simulink library "carnotUIBK_bus"  (R2023b)
settings: Solver=VariableStepAuto  StartTime=0.0  StopTime=10.0  RelTol=1e-3  EnableMultiTasking=on
values from neighbouring files (symbols this model uses):
  A = 7*10*2    (= 140)    [theta_ground_v1.m]    (also in xlswrite1.m = num2cell(data))
  amb_factor = 1    [DOOR.m]    (also in WALL.m; WINDOW.m = 0)
  area = obj.width * obj.height    [DOOR.m]    (also in RES.m = []; ROOM.m = 0; THERMALZONE.m = area + room(kk).area; WALL.m = area - obj.doors(jj).calc_area())
  B = A/(0.5 * P)    (= 8.23529411765)    [theta_ground_v1.m]
  boundary = BOUNDARY()    [BUILDING.m]    (also in WALL.m = '')
  building = obj    [BUILDING.m]    (also in create_building_automatic.m = building.save(); ini_building_automatic.m = building.add_variant_hvac(building.variant_hvac, hvac); load_building_automatic.m = building.save())
  C = zeros(1,length(d)+1)    [CONSTRUCTION.m]    (also in DOOR.m = [0 0 0]; WALL.m = [0 0 0]; WINDOW.m = [0 0 0])
  control = 2    [GAIN.m]    (also in GAINS.m)
  cp = str2num(value)    [CONSTRUCTION.m]
  height = 0    [DOOR.m]    (also in ROOM.m; THERMALZONE.m; WALL.m; WINDOW.m)
  p = [timevec_weather weather(:,12)]    [BOUNDARY.m]    (also in WEATHER.m = 0; init_carnotUIBK.m = cell2mat(carnotUIBKpaths(i,2)))
  rho = str2num(value)    [CONSTRUCTION.m]    (also in theta_ground_v1.m = 2000)
  type = 1    [CONSTRUCTION.m]    (also in GAINS.m = raw_moisture{ii,3}; STRUCTURE.m = 0)
  view_factor = 1    [DOOR.m]    (also in WINDOW.m = 0)
  wall = []    [ROOM.m]
  z = obj.Z    [WALL.m]    (also in theta_ground_v1.m = 0)
  zone = obj.zone(ind)    [THERMALZONE.m]
undefined symbols (not defined in the file or in its folder): const, Dd, get_building, mdot_air, mdot_CO2, mdot_H2O, mdot_VOC, pos, Qdot_C, Qdot_H, Qdot_I_electricity, Qdot_I_light, Qdot_I_person, Qdot_S, Qdot_T_ground, Qdot_T_internal, Qdot_T_neighbour, Qdot_T_opaque, Qdot_T_window, Qdot_V_infiltration, Qdot_V_mech, Qdot_V_window, Qdotc, Qdotr, r_frame, solar_ratio, solar_ratio1, solar_ratio2, Tc, Tr, Ts, Uvalue, wallsurface, window, window_height, window_heigth, window_width, windowsurface, x_CO2, x_H2O, x_VOC
libraries: $bdroot x134, carnot x87, simulink_extras x14, slpidlib x4, simulink x3
(part 7 of 12)

== system carnotUIBK_bus/window/window_TF_shading/alfa_window_in ==
  note: Convective and radiative heat transfer at the INDOOR SURFACE OF A VERTICAL WINDOW
      | with 1-4 layers (each 3 ... 8 mm thick)
  note: WINDOW = FRAME + GLASS
  note: s: surface
      | c: convective
      | r: radiative
  note: CONVENTION:
      | Qdot > 0 and qdots < 0, if Ts > T (heat flows from wall surface to room node),
      | Qdot < 0 and qdots > 0, if Ts < T (heat flows from room node to wall surface).
  note: (W/m^2)
  Ts2 : Inport
  "[sun_t]" : Inport  Port=2
  "[AIV]" : Inport  Port=3
  WDB : Inport  Port=4
  control : Inport  Port=5
  Bus Assignment2 : BusAssignment  AssignedSignals=Qdotc,Qdotr,Qdot_S
  Bus Selector : BusSelector  OutputSignals=Tc,Tr
  Fcn : Fcn  Expr=1.6*(abs(u(1)-u(2)))^0.3
  Fcn1 : Fcn  Expr=(273.15+u(1))^4-(273.15+u(2))^4
  Mux2 : Mux  Inputs=2
  Mux3 : Mux  Inputs=2
  Product : Product  InputSameDT=on  RndMeth=Zero  SaturateOnIntegerOverflow=on  OutDataTypeStr=Inherit: Same as first input
  Product1 : Product  InputSameDT=on  RndMeth=Zero  SaturateOnIntegerOverflow=on  OutDataTypeStr=Inherit: Same as first input
  S_initialize : $bdroot/general/S_initialize  SystemSampleTime=-1  VariantActivationTime=update diagram  AllowFlexibleInterface=on  Latency=0  AutoFrameSizeCalculation=off
  Sum : Sum  Inputs=+-  InputSameDT=on  SaturateOnIntegerOverflow=on  OutDataTypeStr=Inherit: Same as first input
  Sum2 : Sum  Inputs=--+  InputSameDT=on  SaturateOnIntegerOverflow=on  OutDataTypeStr=Inherit: Same as first input
  emission_in : Gain  Gain=emission_in  SaturateOnIntegerOverflow=on  OutDataTypeStr=Inherit: Same as input  ParamDataTypeStr=Inherit: Same as input
  sigma : Constant  Value=5.67e-8
  surface of window glass : Gain  Gain=(1-frame)*windowsurface  SaturateOnIntegerOverflow=on  OutDataTypeStr=Inherit: Same as input  ParamDataTypeStr=Inherit: Same as input
  surface of window1 : Gain  Gain=windowsurface  SaturateOnIntegerOverflow=on  OutDataTypeStr=Inherit: Same as input  ParamDataTypeStr=Inherit: Same as input
  surface of window2 : Gain  Gain=windowsurface  SaturateOnIntegerOverflow=on  OutDataTypeStr=Inherit: Same as input  ParamDataTypeStr=Inherit: Same as input
  transmission_absorption : Subsystem
  view_factor : Gain  Gain=view_factor  SaturateOnIntegerOverflow=on  OutDataTypeStr=Inherit: Same as input  ParamDataTypeStr=Inherit: Same as input
  qdots2 : Outport  VectorParamsAs1DForOutWhenUnconnected=off
  "[S]" : Outport  Port=2  VectorParamsAs1DForOutWhenUnconnected=off
  wires:
  control/1 -> transmission_absorption/3(control)
  WDB/1 -> transmission_absorption/2(WDB)
  transmission_absorption/1(qdot_abs) -> Sum2/3  "qabs"
  transmission_absorption/2(qdot_sol) -> surface of window glass/1  "qdot_sol (>=0)"
  surface of window glass/1 -> Bus Assignment2/4  "Qdot_sol"
  "[sun_t]"/1 -> transmission_absorption/1(sun_t)
  Product/1 -> Sum2/2, surface of window2/1  "qdotr"
  Sum2/1 -> qdots2/1
  emission_in/1 -> view_factor/1
  sigma/1 -> emission_in/1
  Fcn1/1 -> Product/2
  view_factor/1 -> Product/1
  "[AIV]"/1 -> Bus Selector/1
  Mux3/1 -> Fcn1/1
  Bus Selector/2 -> Mux3/2  "<Tr>"
  Fcn/1 -> Product1/2  "hc"
  Mux2/1 -> Fcn/1
  Sum/1 -> Product1/1  "dTc"
  Ts2/1 -> Sum/1, Mux2/1, Mux3/1  "Ts"
  Bus Selector/1 -> Sum/2, Mux2/2  "<Tc>"
  Product1/1 -> surface of window1/1, Sum2/1  "qdotc"
  S_initialize/1 -> Bus Assignment2/1
  surface of window1/1 -> Bus Assignment2/2  "[Qdotc, Qdotr]"
  surface of window2/1 -> Bus Assignment2/3  "[Qdotc, Qdotr]"
  Bus Assignment2/1 -> "[S]"/1

== system carnotUIBK_bus/window/window_TF_shading/alfa_window_out ==
  note: WINDOW = FRAME + GLASS
  note: Convective and radiative heat transfer at the OUTDOOR SURFACE OF A VERTICAL WINDOW
  note: modified
      | weatherdata
  note: s: surface
      | c: convective
      | r: radiative
      | h: in height
      | t: tilted surface
  note: CONVENTION:
      | qdots < 0, if Ts > T, heat flows from window surface (resp. room node) to ambition,
      | qdots > 0, if Ts < T, heat flows from ambition to window surface (resp. room node).
  WDB : Inport
  g : Inport  Port=2
  Ts1 : Inport  Port=3
  Bus Assignment2 : BusAssignment  AssignedSignals=Qdot_T_window
  Bus Selector : BusSelector  OutputSignals=Temperature_Ambient,Temperature_Sky_Radiation,Wind_Speed
  Bus Selector1 : BusSelector  OutputSignals=Incidence_Angle_sun,Solar_Radiation_direct_surface,Solar_Radiation_diffuse_surface
  Mux1 : Mux  Inputs=2
  Mux2 : Mux  Inputs=2
  Product6 : Product  InputSameDT=on  SaturateOnIntegerOverflow=on  OutDataTypeStr=Inherit: Same as first input
  Product7 : Product  InputSameDT=on  SaturateOnIntegerOverflow=on  OutDataTypeStr=Inherit: Same as first input
  Radiation_on_Inclined_Surface : carnot/Weather/Radiation_on_Inclined_Surface  sky=Perez 1990  reflect=0.2
      settings: SourceProductName=Carnot
  S_initialize : $bdroot/general/S_initialize  SystemSampleTime=-1  VariantActivationTime=update diagram  AllowFlexibleInterface=on  Latency=0  AutoFrameSizeCalculation=off
  Sum : Sum  Inputs=+-  InputSameDT=on  SaturateOnIntegerOverflow=on  OutDataTypeStr=Inherit: Same as first input
  Sum2 : Sum  Inputs=+++  InputSameDT=on  SaturateOnIntegerOverflow=on  OutDataTypeStr=Inherit: Same as first input
  Sum3 : Sum  InputSameDT=on  SaturateOnIntegerOverflow=on  OutDataTypeStr=Inherit: Same as first input
  absorption_out * frame : Gain  Gain=absorption_out * frame  SaturateOnIntegerOverflow=on  OutDataTypeStr=Inherit: Same as input  ParamDataTypeStr=Inherit: Same as input
  alfa : Fcn  Expr=3*u(1)+2.8
  position : Constant  Value=pos
  qp rad : Subsystem
  surface of window : Gain  Gain=windowsurface  SaturateOnIntegerOverflow=on  OutDataTypeStr=Inherit: Same as input  ParamDataTypeStr=Inherit: Same as input
  "[sun_t]" : Outport  InitialOutput=0  VectorParamsAs1DForOutWhenUnconnected=off
  qdots1 : Outport  Port=2  InitialOutput=0  VectorParamsAs1DForOutWhenUnconnected=off
  "[S]" : Outport  Port=3  InitialOutput=0  VectorParamsAs1DForOutWhenUnconnected=off
  wires:
  Radiation_on_Inclined_Surface/1 -> Bus Selector1/1
  position/1 -> Radiation_on_Inclined_Surface/2
  Product7/1 -> Sum2/1  "qdot,conv"
  alfa/1 -> Product7/2  "alfa"
  qp rad/1(qprad) -> Sum2/2  "qdotr"
  Ts1/1 -> qp rad/2(Tw), Sum/2  "Ts (outer wall surface)"
  Mux1/1 -> "[sun_t]"/1
  Bus Selector1/2 -> Mux2/1, Sum3/1  "<Solar_Radiation_direct_surface>"
  absorption_out * frame/1 -> Sum2/3
  g/1 -> Product6/2
  Sum2/1 -> surface of window/1, qdots1/1
  Sum3/1 -> absorption_out * frame/1
  Bus Selector1/1 -> Mux1/1  "<Incidence_Angle_sun>"
  WDB/1 -> Radiation_on_Inclined_Surface/1, Bus Selector/1
  Sum/1 -> Product7/1  "dTc"
  Product6/1 -> Mux1/2
  Mux2/1 -> Product6/1
  Bus Selector1/3 -> Mux2/2, Sum3/2  "<Solar_Radiation_diffuse_surface>"
  Bus Selector/1 -> qp rad/1(Ta), Sum/1  "<Temperature_Ambient>"
  Bus Selector/2 -> qp rad/3(Tsky)  "<Temperature_Sky_Radiation>"
  Bus Selector/3 -> alfa/1  "<Wind_Speed>"
  Bus Assignment2/1 -> "[S]"/1
  surface of window/1 -> Bus Assignment2/2
  S_initialize/1 -> Bus Assignment2/1

== system carnotUIBK_bus/window/window_TF_shading/lambda_window ==
  note: Heat conduction in a window (ONLY SURFACE LAYER CONNECTABLE)
  note: Timeconstant of window is calculated
      | in the mask initialization
  qdots1 : Inport
  qdots2 : Inport  Port=2
  Product1 : Product  InputSameDT=on  RndMeth=Zero  SaturateOnIntegerOverflow=on  OutDataTypeStr=Inherit: Same as first input
  Product6 : Product  InputSameDT=on  RndMeth=Zero  SaturateOnIntegerOverflow=on  OutDataTypeStr=Inherit: Same as first input
  R_win : Constant  Value=Rwin
  Sum1 : Sum  InputSameDT=on  SaturateOnIntegerOverflow=on  OutDataTypeStr=Inherit: Same as first input
  Sum3 : Sum  InputSameDT=on  SaturateOnIntegerOverflow=on  OutDataTypeStr=Inherit: Same as first input
  Transfer Fcn : TransferFcn  Denominator=[timeconst 1]
  Transfer Fcn1 : TransferFcn  Denominator=[timeconst 1]
  Ts1 : Outport  VectorParamsAs1DForOutWhenUnconnected=off
  Ts2 : Outport  Port=2  VectorParamsAs1DForOutWhenUnconnected=off
  wires:
  Transfer Fcn1/1 -> Ts2/1, Sum3/2
  Transfer Fcn/1 -> Ts1/1, Sum1/2
  qdots1/1 -> Product6/2
  qdots2/1 -> Product1/2
  Product6/1 -> Sum3/1
  Sum3/1 -> Transfer Fcn/1
  Product1/1 -> Sum1/1
  Sum1/1 -> Transfer Fcn1/1
  R_win/1 -> Product6/1, Product1/1  "R_win"

== system carnotUIBK_bus/HVAC/HVAC_1001_electrical heaters/electrical heater zone 1/Transfer Fcn (with initial states) ==
  In1 : Inport
  State Space : StateSpace  A=A  B=B  C=C  D=Dd  InitialCondition=X0
  Out1 : Outport  InitialOutput=0  VectorParamsAs1DForOutWhenUnconnected=off
  wires:
  In1/1 -> State Space/1
  State Space/1 -> Out1/1

== system carnotUIBK_bus/HVAC/HVAC_2001_ventilation system simple/ventilation_zone 1/Subsystem ==
  note: (kg/s)
  note: (kg/s)
  note: (kg/s)
  note: (kg/kg)
  note: (kg/kg)
  note: ASSUMPTION: mdot_air_out2in = mdot_air_in2out !
  mdot_air : Inport
  x_in : Inport  Port=2
  x_out : Inport  Port=3
  Demux2 : Demux  Outputs=2
      settings: DisplayOption=none
  Demux3 : Demux  Outputs=2
      settings: DisplayOption=none
  Fcn{,1..3} (4 alike) : Fcn  Expr=u / (1+u)
  Product5 : Product  InputSameDT=on  SaturateOnIntegerOverflow=on  OutDataTypeStr=Inherit: Same as first input
  Product6 : Product  InputSameDT=on  SaturateOnIntegerOverflow=on  OutDataTypeStr=Inherit: Same as first input
  Sum1 : Sum  Inputs=+-  InputSameDT=on  SaturateOnIntegerOverflow=on  OutDataTypeStr=Inherit: Same as first input
  Sum2 : Sum  Inputs=+-  InputSameDT=on  SaturateOnIntegerOverflow=on  OutDataTypeStr=Inherit: Same as first input
  mdot_H2O : Outport  VectorParamsAs1DForOutWhenUnconnected=off
  mdot_CO2 : Outport  Port=2  VectorParamsAs1DForOutWhenUnconnected=off
  wires:
  x_out/1 -> Demux2/1
  Demux2/1 -> Fcn/1  "x_H2O_out"
  Demux2/2 -> Fcn1/1  "x_CO2_out"
  Demux3/2 -> Fcn3/1  "x_CO2_in"
  Demux3/1 -> Fcn2/1  "x_H2O_in"
  x_in/1 -> Demux3/1
  Fcn/1 -> Sum1/1
  Fcn2/1 -> Sum1/2
  Fcn1/1 -> Sum2/1
  Fcn3/1 -> Sum2/2
  Sum2/1 -> Product6/2
  Sum1/1 -> Product5/2
  mdot_air/1 -> Product6/1, Product5/1  "mdot_air >=0"
  Product6/1 -> mdot_CO2/1
  Product5/1 -> mdot_H2O/1

== system carnotUIBK_bus/HVAC/HVAC_9002_window opening/window opening 1/Transfer Fcn (with initial states) ==
  In1 : Inport
  State Space : StateSpace  A=A  B=B  C=C  D=Dd  InitialCondition=X0
  Out1 : Outport  InitialOutput=0  VectorParamsAs1DForOutWhenUnconnected=off
  wires:
  In1/1 -> State Space/1
  State Space/1 -> Out1/1

== system carnotUIBK_bus/HVAC/HVAC_9002_window opening/window opening 1/Transfer Fcn (with initial states)1 ==
  In1 : Inport
  State Space : StateSpace  A=A  B=B  C=C  D=Dd  InitialCondition=X0
  Out1 : Outport  InitialOutput=0  VectorParamsAs1DForOutWhenUnconnected=off
  wires:
  State Space/1 -> Out1/1
  In1/1 -> State Space/1

== system carnotUIBK_bus/HVAC/HVAC_9002_window opening/window opening 1/Transfer Fcn (with initial states)2 ==
  In1 : Inport
  State Space : StateSpace  A=A  B=B  C=C  D=Dd  InitialCondition=X0
  Out1 : Outport  InitialOutput=0  VectorParamsAs1DForOutWhenUnconnected=off
  wires:
  In1/1 -> State Space/1
  State Space/1 -> Out1/1

== system carnotUIBK_bus/HVAC/HVAC_9002_window opening/window opening 2/Transfer Fcn (with initial states)1 ==
  In1 : Inport
  State Space : StateSpace  A=A  B=B  C=C  D=Dd  InitialCondition=X0
  Out1 : Outport  InitialOutput=0  VectorParamsAs1DForOutWhenUnconnected=off
  wires:
  State Space/1 -> Out1/1
  In1/1 -> State Space/1

== system carnotUIBK_bus/HVAC/HVAC_9002_window opening/window opening 2/Transfer Fcn (with initial states)2 ==
  In1 : Inport
  State Space : StateSpace  A=A  B=B  C=C  D=Dd  InitialCondition=X0
  Out1 : Outport  InitialOutput=0  VectorParamsAs1DForOutWhenUnconnected=off
  wires:
  In1/1 -> State Space/1
  State Space/1 -> Out1/1

== system carnotUIBK_bus/HVAC/HVAC_9002_window opening/window opening 2/Transfer Fcn (with initial states)3 ==
  In1 : Inport
  State Space : StateSpace  A=A  B=B  C=C  D=Dd  InitialCondition=X0
  Out1 : Outport  InitialOutput=0  VectorParamsAs1DForOutWhenUnconnected=off
  wires:
  In1/1 -> State Space/1
  State Space/1 -> Out1/1

== system carnotUIBK_bus/HVAC/HVAC_9002_window opening/window opening 3/Transfer Fcn (with initial states)1 ==
  In1 : Inport
  State Space : StateSpace  A=A  B=B  C=C  D=Dd  InitialCondition=X0
  Out1 : Outport  InitialOutput=0  VectorParamsAs1DForOutWhenUnconnected=off
  wires:
  State Space/1 -> Out1/1
  In1/1 -> State Space/1

== system carnotUIBK_bus/HVAC/HVAC_9002_window opening/window opening 3/Transfer Fcn (with initial states)2 ==
  In1 : Inport
  State Space : StateSpace  A=A  B=B  C=C  D=Dd  InitialCondition=X0
  Out1 : Outport  InitialOutput=0  VectorParamsAs1DForOutWhenUnconnected=off
  wires:
  In1/1 -> State Space/1
  State Space/1 -> Out1/1

== system carnotUIBK_bus/HVAC/HVAC_9002_window opening/window opening 3/Transfer Fcn (with initial states)3 ==
  In1 : Inport
  State Space : StateSpace  A=A  B=B  C=C  D=Dd  InitialCondition=X0
  Out1 : Outport  InitialOutput=0  VectorParamsAs1DForOutWhenUnconnected=off
  wires:
  In1/1 -> State Space/1
  State Space/1 -> Out1/1

== system carnotUIBK_bus/HVAC/HVAC_9002_window opening/window opening 4/Transfer Fcn (with initial states)1 ==
  In1 : Inport
  State Space : StateSpace  A=A  B=B  C=C  D=Dd  InitialCondition=X0
  Out1 : Outport  InitialOutput=0  VectorParamsAs1DForOutWhenUnconnected=off
  wires:
  State Space/1 -> Out1/1
  In1/1 -> State Space/1

== system carnotUIBK_bus/HVAC/HVAC_9002_window opening/window opening 4/Transfer Fcn (with initial states)2 ==
  In1 : Inport
  State Space : StateSpace  A=A  B=B  C=C  D=Dd  InitialCondition=X0
  Out1 : Outport  InitialOutput=0  VectorParamsAs1DForOutWhenUnconnected=off
  wires:
  In1/1 -> State Space/1
  State Space/1 -> Out1/1

== system carnotUIBK_bus/HVAC/HVAC_9002_window opening/window opening 4/Transfer Fcn (with initial states)3 ==
  In1 : Inport
  State Space : StateSpace  A=A  B=B  C=C  D=Dd  InitialCondition=X0
  Out1 : Outport  InitialOutput=0  VectorParamsAs1DForOutWhenUnconnected=off
  wires:
  In1/1 -> State Space/1
  State Space/1 -> Out1/1

== system carnotUIBK_bus/HVAC/HVAC_9002_window opening/window opening 5/Transfer Fcn (with initial states)1 ==
  In1 : Inport
  State Space : StateSpace  A=A  B=B  C=C  D=Dd  InitialCondition=X0
  Out1 : Outport  InitialOutput=0  VectorParamsAs1DForOutWhenUnconnected=off
  wires:
  State Space/1 -> Out1/1
  In1/1 -> State Space/1

== system carnotUIBK_bus/HVAC/HVAC_9002_window opening/window opening 5/Transfer Fcn (with initial states)2 ==
  In1 : Inport
  State Space : StateSpace  A=A  B=B  C=C  D=Dd  InitialCondition=X0
  Out1 : Outport  InitialOutput=0  VectorParamsAs1DForOutWhenUnconnected=off
  wires:
  In1/1 -> State Space/1
  State Space/1 -> Out1/1

== system carnotUIBK_bus/HVAC/HVAC_9002_window opening/window opening 5/Transfer Fcn (with initial states)3 ==
  In1 : Inport
  State Space : StateSpace  A=A  B=B  C=C  D=Dd  InitialCondition=X0
  Out1 : Outport  InitialOutput=0  VectorParamsAs1DForOutWhenUnconnected=off
  wires:
  In1/1 -> State Space/1
  State Space/1 -> Out1/1

== system carnotUIBK_bus/HVAC/HVAC_9002_window opening/window opening 6/Transfer Fcn (with initial states)1 ==
  In1 : Inport
  State Space : StateSpace  A=A  B=B  C=C  D=Dd  InitialCondition=X0
  Out1 : Outport  InitialOutput=0  VectorParamsAs1DForOutWhenUnconnected=off
  wires:
  State Space/1 -> Out1/1
  In1/1 -> State Space/1

== system carnotUIBK_bus/HVAC/HVAC_9002_window opening/window opening 6/Transfer Fcn (with initial states)2 ==
  In1 : Inport
  State Space : StateSpace  A=A  B=B  C=C  D=Dd  InitialCondition=X0
  Out1 : Outport  InitialOutput=0  VectorParamsAs1DForOutWhenUnconnected=off
  wires:
  In1/1 -> State Space/1
  State Space/1 -> Out1/1

== system carnotUIBK_bus/HVAC/HVAC_9002_window opening/window opening 6/Transfer Fcn (with initial states)3 ==
  In1 : Inport
  State Space : StateSpace  A=A  B=B  C=C  D=Dd  InitialCondition=X0
  Out1 : Outport  InitialOutput=0  VectorParamsAs1DForOutWhenUnconnected=off
  wires:
  In1/1 -> State Space/1
  State Space/1 -> Out1/1

== system carnotUIBK_bus/gain/People/W//ppl (activity)/LUT_Qdot_dry ==
  note: SENSITIVE/DRY HEAT POWER emitted from a person in a room
  activity : Inport
  Top : Inport  Port=2
  Look-Up Table Qdot_dry : Subsystem  mask(Lookup Table (2-D)){x=[10 12 14 16 18 20 22 23 24 25 26 28 30 32 34], y=[0 1 2 3 4], t=[135 135 135 170 210; 125 125 125 160 195; 115 115 115 150 180; 105 105 105 135 165; 100 100 100 125 152; 95 95 95 115 140; 90 90 90 105 125; 85 85 85 100 117; 80 80 80 95 110; 75 75 75 90 102; 70 70 70 85 95; 60 60 60 70 80; 50 50 50 60 65; 30 30 30 35 40; 0 0 0 0 0]}
      mask prompts: x "Row:"; y "Column:"; t "Table:"
      mask help: Performs 2-D linear interpolation of input values using the specified input/output table. Extrapolation is performed outside the table boundaries.
      mask init:
      | [r,c]=size(t);
      | x=reshape(x,prod(size(x)),1);
      | xi=x(:,ones(1,c));
      | minx=min(x); maxx=max(x);
      | mint=min(min(t)); maxt=max(max(t));
      mask Display: plot(xi,t,[minx maxx],[mint mint],[minx minx],[mint maxt])
  Qdot_dry : Outport  InitialOutput=0  VectorParamsAs1DForOutWhenUnconnected=off
  wires:
  activity/1 -> Look-Up Table Qdot_dry/2(Cols)
  Look-Up Table Qdot_dry/1(U) -> Qdot_dry/1
  Top/1 -> Look-Up Table Qdot_dry/1(Rows)

== system carnotUIBK_bus/gain/People/W//ppl (activity)/LUT_Qdot_hum1 ==
  note: LATENT/HUMID HEAT POWER emitted from a person in a room
  activity : Inport
  Top : Inport  Port=2
  Look-Up Table Qdot_hum : Subsystem  mask(Lookup Table (2-D)){x=[10 12 14 16 18 20 22 23 24 25 26 28 30 32 34], y=[0 1 2 3 4], t=[20 20 20 55 100; 20 20 20 55 100; 20 20 20 55 100; 21 21 21 58 105; 23 23 23 65 115; 25 25 25 75 130; 30 30 30 85 145; 35 35 35 90 155; 40 40 40 95 160; 45 45 45 100 167; 50 50 50 105 175; 60 60 60 115 190; 70 70 70 125 205; 80 80 80 135 225; 90 90 90 145 245]}
      mask prompts: x "Row:"; y "Column:"; t "Table:"
      mask help: Performs 2-D linear interpolation of input values using the specified input/output table. Extrapolation is performed outside the table boundaries.
      mask init:
      | [r,c]=size(t);
      | x=reshape(x,prod(size(x)),1);
      | xi=x(:,ones(1,c));
      | minx=min(x); maxx=max(x);
      | mint=min(min(t)); maxt=max(max(t));
      mask Display: plot(xi,t,[minx maxx],[mint mint],[minx minx],[mint maxt])
  Qdot_hum : Outport  InitialOutput=0  VectorParamsAs1DForOutWhenUnconnected=off
  wires:
  Top/1 -> Look-Up Table Qdot_hum/1(Rows)
  activity/1 -> Look-Up Table Qdot_hum/2(Cols)
  Look-Up Table Qdot_hum/1(U) -> Qdot_hum/1

== system carnotUIBK_bus/gain/People/W//ppl (activity)/LUT_mdot_CO2 ==
  note: CO2 MASS FLOW emitted from a person in a room
  activity : Inport
  Look-Up mdot_CO2 : Lookup  InputValues=[0 1 2 3 4]  Table=[0.567 0.708 1.133 2.031 3.305]*10^-5
  mdot_CO2 : Outport  InitialOutput=0  VectorParamsAs1DForOutWhenUnconnected=off
  wires:
  Look-Up mdot_CO2/1 -> mdot_CO2/1
  activity/1 -> Look-Up mdot_CO2/1

== system carnotUIBK_bus/gain/People/W//ppl (activity)/LUT_mdot_H2O ==
  note: WATER MASS FLOW emitted from a person in a room
  activity : Inport
  Top : Inport  Port=2
  Look-Up Table mdot_H2O : Subsystem  mask(Lookup Table (2-D)){x=[10 12 14 16 18 20 22 23 24 25 26 32], y=[0 1 2 3 4], t=[30 30 30 90 150; 30 30 30 90 150; 30 30 30 90 150; 30 30 30 90 155; 35 35 35 95 165; 40 40 40 110 185; 45 45 45 125 200; 50 50 50 130 210; 55 55 55 130 225; 60 60 60 140 240; 65 65 65 150 270; 120 120 120 250 450]/(3.6*1e6)}
      mask prompts: x "Row:"; y "Column:"; t "Table:"
      mask help: Performs 2-D linear interpolation of input values using the specified input/output table. Extrapolation is performed outside the table boundaries.
      mask init:
      | [r,c]=size(t);
      | x=reshape(x,prod(size(x)),1);
      | xi=x(:,ones(1,c));
      | minx=min(x); maxx=max(x);
      | mint=min(min(t)); maxt=max(max(t));
      mask Display: plot(xi,t,[minx maxx],[mint mint],[minx minx],[mint maxt])
  mdot_H2O : Outport  InitialOutput=0  VectorParamsAs1DForOutWhenUnconnected=off
  wires:
  Look-Up Table mdot_H2O/1(U) -> mdot_H2O/1
  activity/1 -> Look-Up Table mdot_H2O/2(Cols)
  Top/1 -> Look-Up Table mdot_H2O/1(Rows)

== system carnotUIBK_bus/gain/People/W//ppl (constant)/LUT_mdot_CO2 ==
  note: CO2 MASS FLOW emitted from a person in a room
  activity : Inport
  Look-Up mdot_CO2 : Lookup  InputValues=[0 1 2 3 4]  Table=[0.567 0.708 1.133 2.031 3.305]*10^-5
  mdot_CO2 : Outport  InitialOutput=0  VectorParamsAs1DForOutWhenUnconnected=off
  wires:
  Look-Up mdot_CO2/1 -> mdot_CO2/1
  activity/1 -> Look-Up mdot_CO2/1

== system carnotUIBK_bus/gain/People/W//ppl (constant)/LUT_mdot_H2O ==
  note: WATER MASS FLOW emitted from a person in a room
  activity : Inport
  Top : Inport  Port=2
  Look-Up Table mdot_H2O : Subsystem  mask(Lookup Table (2-D)){x=[10 12 14 16 18 20 22 23 24 25 26 32], y=[0 1 2 3 4], t=[30 30 30 90 150; 30 30 30 90 150; 30 30 30 90 150; 30 30 30 90 155; 35 35 35 95 165; 40 40 40 110 185; 45 45 45 125 200; 50 50 50 130 210; 55 55 55 130 225; 60 60 60 140 240; 65 65 65 150 270; 120 120 120 250 450]/(3.6*1e6)}
      mask prompts: x "Row:"; y "Column:"; t "Table:"
      mask help: Performs 2-D linear interpolation of input values using the specified input/output table. Extrapolation is performed outside the table boundaries.
      mask init:
      | [r,c]=size(t);
      | x=reshape(x,prod(size(x)),1);
      | xi=x(:,ones(1,c));
      | minx=min(x); maxx=max(x);
      | mint=min(min(t)); maxt=max(max(t));
      mask Display: plot(xi,t,[minx maxx],[mint mint],[minx minx],[mint maxt])
  mdot_H2O : Outport  InitialOutput=0  VectorParamsAs1DForOutWhenUnconnected=off
  wires:
  Look-Up Table mdot_H2O/1(U) -> mdot_H2O/1
  activity/1 -> Look-Up Table mdot_H2O/2(Cols)
  Top/1 -> Look-Up Table mdot_H2O/1(Rows)

== system carnotUIBK_bus/infiltration/infiltration_pressure/infiltration_pressure/dP_infiltration ==
  T_int : Inport
  T_ext : Inport  Port=2
  windspeed : Inport  Port=3
  wind_angle : Inport  Port=4
  air_density_ext : Inport  Port=5
  H_window : Inport  Port=6
  add_coeff_wind : Inport  Port=7
  facade_angle : Inport  Port=8
  Add : Sum
  Add1 : Sum
  Divide : Product  Inputs=/****
  Gain : Gain  Gain=0.5
  K : Constant  Value=273.15
  Product : Product
  Product1 : Product  Inputs=3
  Sum : Sum  Inputs=|+-
  calculate wind_coeff : Subsystem
  g : Constant  Value=9.81
  half of window height : Gain  Gain=0.5
  dP_total : Outport  VectorParamsAs1DForOutWhenUnconnected=off
  wires:
  T_int/1 -> Add1/2, Sum/1
  T_ext/1 -> Sum/2
  Sum/1 -> Divide/2  "delta_T"
  air_density_ext/1 -> Product1/1, Divide/4
  Product/1 -> Gain/1
  Gain/1 -> Product1/3
  Add/1 -> dP_total/1
  g/1 -> Divide/3
  half of window height/1 -> Divide/5
  H_window/1 -> half of window height/1
  wind_angle/1 -> calculate wind_coeff/1(wind_angle)
  calculate wind_coeff/1(wind_coeff) -> Product1/2
  add_coeff_wind/1 -> calculate wind_coeff/2(additional_coeff_wind)
  facade_angle/1 -> calculate wind_coeff/3(facade_angle)
  Product1/1 -> Add/2
  windspeed/1 -> Product/1, Product/2
  Divide/1 -> Add/1
  K/1 -> Add1/1
  Add1/1 -> Divide/1

== system carnotUIBK_bus/infiltration/infiltration_pressure/infiltration_pressure/power_law_infiltration ==
  dP : Inport
  C : Inport  Port=2
  n : Inport  Port=3
  density : Inport  Port=4
  1/3600 : Gain  Gain=1/3600
  Product2 : Product
  Product4 : Product
  abs : Abs  SaturateOnIntegerOverflow=off
  pow_law : Math  Operator=pow  SignedPower=on
  m_dot : Outport  VectorParamsAs1DForOutWhenUnconnected=off
  wires:
  pow_law/1 -> Product2/1
  C/1 -> 1/3600/1
  Product2/1 -> Product4/1
  n/1 -> pow_law/2
  dP/1 -> abs/1
  density/1 -> Product4/2
  Product4/1 -> m_dot/1
  1/3600/1 -> Product2/2
  abs/1 -> pow_law/1

== system carnotUIBK_bus/room_node/1-node/pressure/Subsystem ==
  note: (J/(kg*K)
  T : Inport
  Celsius2Kelvin : Bias  Bias=273.15  SaturateOnIntegerOverflow=off
  air_gas_constant : Gain  Gain=287  SaturateOnIntegerOverflow=on  OutDataTypeStr=Inherit: Same as input  ParamDataTypeStr=Inherit: Same as input
  R*T ' : Outport  VectorParamsAs1DForOutWhenUnconnected=off
  wires:
  Celsius2Kelvin/1 -> air_gas_constant/1
  T/1 -> Celsius2Kelvin/1
  air_gas_constant/1 -> R*T '/1

== system carnotUIBK_bus/room_node/1-node/pressure/Transfer Fcn (with initial outputs)1 ==
  In1 : Inport
  State Space : StateSpace  A=A  B=B  C=C  D=Dd  InitialCondition=X0
  Out1 : Outport  InitialOutput=0  VectorParamsAs1DForOutWhenUnconnected=off
  wires:
  State Space/1 -> Out1/1
  In1/1 -> State Space/1

== system carnotUIBK_bus/room_node/2-node/density and capacity/Transfer Fcn (with initial outputs) ==
  In1 : Inport
  State Space : StateSpace  A=A  B=B  C=C  D=Dd  InitialCondition=X0
  Out1 : Outport  InitialOutput=0  VectorParamsAs1DForOutWhenUnconnected=off
  wires:
  In1/1 -> State Space/1
  State Space/1 -> Out1/1

== system carnotUIBK_bus/room_node/2-node/pressure/Subsystem ==
  note: (J/(kg*K)
  T : Inport
  Celsius2Kelvin : Bias  Bias=273.15  SaturateOnIntegerOverflow=off
  air_gas_constant : Gain  Gain=287  SaturateOnIntegerOverflow=on  OutDataTypeStr=Inherit: Same as input  ParamDataTypeStr=Inherit: Same as input
  R*T ' : Outport  VectorParamsAs1DForOutWhenUnconnected=off
  wires:
  Celsius2Kelvin/1 -> air_gas_constant/1
  T/1 -> Celsius2Kelvin/1
  air_gas_constant/1 -> R*T '/1

== system carnotUIBK_bus/room_node/2-node/pressure/Transfer Fcn (with initial outputs)1 ==
  In1 : Inport
  State Space : StateSpace  A=A  B=B  C=C  D=Dd  InitialCondition=X0
  Out1 : Outport  InitialOutput=0  VectorParamsAs1DForOutWhenUnconnected=off
  wires:
  State Space/1 -> Out1/1
  In1/1 -> State Space/1

== system carnotUIBK_bus/room_node/2-node_ideal/pressure/Subsystem ==
  note: (J/(kg*K)
  T : Inport
  Celsius2Kelvin : Bias  Bias=273.15  SaturateOnIntegerOverflow=off
  air_gas_constant : Gain  Gain=287  SaturateOnIntegerOverflow=on  OutDataTypeStr=Inherit: Same as input  ParamDataTypeStr=Inherit: Same as input
  R*T ' : Outport  VectorParamsAs1DForOutWhenUnconnected=off
  wires:
  Celsius2Kelvin/1 -> air_gas_constant/1
  T/1 -> Celsius2Kelvin/1
  air_gas_constant/1 -> R*T '/1

== system carnotUIBK_bus/room_node/2-node_ideal/pressure/Transfer Fcn (with initial outputs)1 ==
  In1 : Inport
  State Space : StateSpace  A=A  B=B  C=C  D=Dd  InitialCondition=X0
  Out1 : Outport  InitialOutput=0  VectorParamsAs1DForOutWhenUnconnected=off
  wires:
  State Space/1 -> Out1/1
  In1/1 -> State Space/1

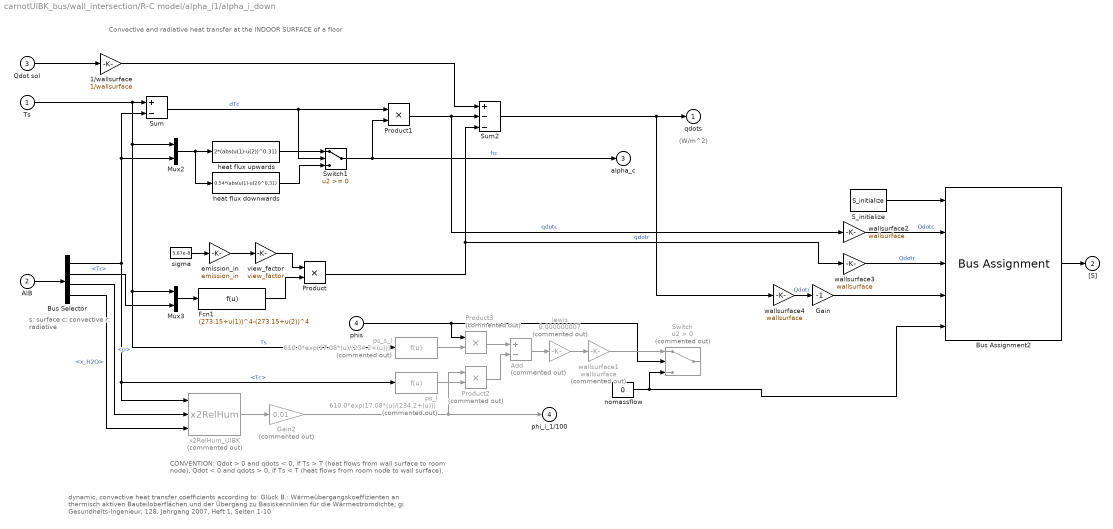
== system carnotUIBK_bus/wall_intersection/R-C model/alpha_i1/alpha_i_down ==
  note: dynamic, convective heat transfer coefficients according to: Glück B.: Wärmeübergangskoeffizienten an thermisch aktiven Bauteiloberflächen
      | und der Übergang zu Basiskennlinien für die Wärmestromdichte; gi Gesundheits-Ingenieur; 128. Jahrgang 2007, Heft 1, Seiten 1-10
  note: s: surface
      | c: convective
      | r: radiative
  note: CONVENTION:
      | Qdot > 0 and qdots < 0, if Ts > T (heat flows from wall surface to room node),
      | Qdot < 0 and qdots > 0, if Ts < T (heat flows from room node to wall surface).
  note: Convective and radiative heat transfer at the INDOOR SURFACE of a floor
  note: (W/m^2)
  Ts : Inport
  AIB : Inport  Port=2
  Qdot sol : Inport  Port=3
  phis : Inport  Port=4
  1/wallsurface : Gain  Gain=1/wallsurface  SaturateOnIntegerOverflow=on  OutDataTypeStr=Inherit: Same as input  ParamDataTypeStr=Inherit: Same as input
  Add : Sum  Commented=on  Inputs=+-
  Bus Assignment2 : BusAssignment  AssignedSignals=Qdotc,Qdotr,Qdot_T_neighbour,mdot_H2O
  Bus Selector : BusSelector  OutputSignals=Tc,Tr,p,x_H2O
  Fcn1 : Fcn  Expr=(273.15+u(1))^4-(273.15+u(2))^4
  Gain : Gain  Gain=-1
  Gain2 : Gain  Commented=on  Gain=0.01
  Mux2 : Mux  Inputs=2
  Mux3 : Mux  Inputs=2
  Product : Product  InputSameDT=on  RndMeth=Zero  SaturateOnIntegerOverflow=on  OutDataTypeStr=Inherit: Same as first input
  Product1 : Product  InputSameDT=on  RndMeth=Zero  SaturateOnIntegerOverflow=on  OutDataTypeStr=Inherit: Same as first input
  Product2 : Product  Commented=on  RndMeth=Zero
  Product3 : Product  Commented=on  RndMeth=Zero
  S_initialize : $bdroot/general/S_initialize  SystemSampleTime=-1  VariantActivationTime=update diagram  AllowFlexibleInterface=on  Latency=0  AutoFrameSizeCalculation=off
  Sum : Sum  Inputs=+-  InputSameDT=on  SaturateOnIntegerOverflow=on  OutDataTypeStr=Inherit: Same as first input
  Sum2 : Sum  Inputs=+--  InputSameDT=on  SaturateOnIntegerOverflow=on  OutDataTypeStr=Inherit: Same as first input
  Switch : Switch  Commented=on  Criteria=u2 > Threshold  SaturateOnIntegerOverflow=off  InputSameDT=off
  Switch1 : Switch  SaturateOnIntegerOverflow=off  InputSameDT=off
  emission_in : Gain  Gain=emission_in  SaturateOnIntegerOverflow=on  OutDataTypeStr=Inherit: Same as input  ParamDataTypeStr=Inherit: Same as input
  heat flux downwards : Fcn  Expr=0.54*(abs(u(1)-u(2))^0.31)
  heat flux upwards : Fcn  Expr=2*(abs(u(1)-u(2))^0.31)
  lewis : Gain  Commented=on  Gain=0.000000007  SaturateOnIntegerOverflow=on  OutDataTypeStr=Inherit: Same as input  ParamDataTypeStr=Inherit: Same as input
  nomassflow : Constant  Value=0
  ps_l : Fcn  Commented=on  Expr=610.0*exp(17.08*(u)/(234.2+(u)))
  ps_s_l : Fcn  Commented=on  Expr=610.0*exp(17.08*(u)/(234.2+(u)))
  sigma : Constant  Value=5.67e-8
  view_factor : Gain  Gain=view_factor  SaturateOnIntegerOverflow=on  OutDataTypeStr=Inherit: Same as input  ParamDataTypeStr=Inherit: Same as input
  wallsurface1 : Gain  Commented=on  Gain=wallsurface  SaturateOnIntegerOverflow=on  OutDataTypeStr=Inherit: Same as input  ParamDataTypeStr=Inherit: Same as input
  wallsurface2 : Gain  Gain=wallsurface  SaturateOnIntegerOverflow=on  OutDataTypeStr=Inherit: Same as input  ParamDataTypeStr=Inherit: Same as input
  wallsurface3 : Gain  Gain=wallsurface  SaturateOnIntegerOverflow=on  OutDataTypeStr=Inherit: Same as input  ParamDataTypeStr=Inherit: Same as input
  wallsurface4 : Gain  Gain=wallsurface  SaturateOnIntegerOverflow=on  OutDataTypeStr=Inherit: Same as input  ParamDataTypeStr=Inherit: Same as input
  x2RelHum_UIBK : carnot/Basic/Material_Properties/x2RelHum  Commented=on
      settings: SourceProductName=Carnot
  qdots : Outport  InitialOutput=0  VectorParamsAs1DForOutWhenUnconnected=off
  "[S]" : Outport  Port=2  InitialOutput=0  VectorParamsAs1DForOutWhenUnconnected=off
  alpha_c : Outport  Port=3  InitialOutput=0  VectorParamsAs1DForOutWhenUnconnected=off
  phi_i_1/100 : Outport  Port=4  InitialOutput=0  VectorParamsAs1DForOutWhenUnconnected=off
  wires:
  heat flux downwards/1 -> Switch1/3
  heat flux upwards/1 -> Switch1/1
  Sum/1 -> Product1/1, Switch1/2  "dTc"
  1/wallsurface/1 -> Sum2/1
  Switch1/1 -> alpha_c/1, Product1/2  "hc"
  Product1/1 -> wallsurface2/1, Sum2/2  "qdotc"
  Mux2/1 -> heat flux upwards/1, heat flux downwards/1
  Bus Selector/2 -> Mux3/2  "<Tr>"
  Ts/1 -> Mux2/1, Mux3/1, ps_s_l/1, Sum/1  "Ts"
  ? -> ?
  Product/1 -> wallsurface3/1, Sum2/3  "qdotr"
  emission_in/1 -> view_factor/1
  Bus Selector/1 -> x2RelHum_UIBK/1, ps_l/1, Mux2/2, Sum/2  "<Tc>"
  AIB/1 -> Bus Selector/1
  Sum2/1 -> wallsurface4/1, qdots/1
  sigma/1 -> emission_in/1
  Mux3/1 -> Fcn1/1
  Fcn1/1 -> Product/2
  x2RelHum_UIBK/1 -> Gain2/1
  Bus Selector/3 -> x2RelHum_UIBK/2  "<p>"
  Bus Selector/4 -> x2RelHum_UIBK/3  "<x_H2O>"
  Gain2/1 -> phi_i_1/100/1, Product2/1
  lewis/1 -> wallsurface1/1
  ps_l/1 -> Product2/2
  ps_s_l/1 -> Product3/2
  Product3/1 -> Add/1
  Product2/1 -> Add/2
  Add/1 -> lewis/1
  phis/1 -> Switch/2, Product3/1
  view_factor/1 -> Product/1
  wallsurface1/1 -> Switch/1
  nomassflow/1 -> Bus Assignment2/5, Switch/3
  Qdot sol/1 -> 1/wallsurface/1
  wallsurface3/1 -> Bus Assignment2/3  "Qdotr"
  wallsurface2/1 -> Bus Assignment2/2  "Qdotc"
  S_initialize/1 -> Bus Assignment2/1
  Bus Assignment2/1 -> "[S]"/1
  wallsurface4/1 -> Gain/1  "Qdotr"
  Gain/1 -> Bus Assignment2/4

== system carnotUIBK_bus/wall_intersection/R-C model/alpha_i1/alpha_i_horizontal ==
  note: dynamic, convective heat transfer coefficients according to: Glück B.: Wärmeübergangskoeffizienten an thermisch aktiven Bauteiloberflächen
      | und der Übergang zu Basiskennlinien für die Wärmestromdichte; gi Gesundheits-Ingenieur; 128. Jahrgang 2007, Heft 1, Seiten 1-10
  note: s: surface
      | c: convective
      | r: radiative
  note: CONVENTION:
      | Qdot > 0 and qdots < 0, if Ts > T (heat flows from wall surface to room node),
      | Qdot < 0 and qdots > 0, if Ts < T (heat flows from room node to wall surface).
  note: Convective and radiative heat transfer at the INDOOR SURFACE of a VERTICAL OUTER WALL
  note: (W/m^2)
  Ts : Inport
  AIB : Inport  Port=2
  Qdot sol : Inport  Port=3
  phis : Inport  Port=4
  1/wallsurface : Gain  Gain=1/wallsurface  SaturateOnIntegerOverflow=on  OutDataTypeStr=Inherit: Same as input  ParamDataTypeStr=Inherit: Same as input
  Add : Sum  Commented=on  Inputs=+-
  Bus Assignment2 : BusAssignment  AssignedSignals=Qdotc,Qdotr,Qdot_T_neighbour,mdot_H2O
  Bus Selector : BusSelector  OutputSignals=Tc,Tr,p,x_H2O
  Fcn : Fcn  Expr=1.6*(abs(u(1)-u(2)))^0.3
  Fcn1 : Fcn  Expr=(273.15+u(1))^4-(273.15+u(2))^4
  Gain2 : Gain  Commented=on  Gain=0.01
  Mux2 : Mux  Inputs=2
  Mux3 : Mux  Inputs=2
  Product : Product  InputSameDT=on  RndMeth=Zero  SaturateOnIntegerOverflow=on  OutDataTypeStr=Inherit: Same as first input
  Product1 : Product  InputSameDT=on  RndMeth=Zero  SaturateOnIntegerOverflow=on  OutDataTypeStr=Inherit: Same as first input
  Product2 : Product  Commented=on  RndMeth=Zero
  Product3 : Product  Commented=on  RndMeth=Zero
  S_initialize : $bdroot/general/S_initialize  SystemSampleTime=-1  VariantActivationTime=update diagram  AllowFlexibleInterface=on  Latency=0  AutoFrameSizeCalculation=off
  Sum : Sum  Inputs=+-  InputSameDT=on  SaturateOnIntegerOverflow=on  OutDataTypeStr=Inherit: Same as first input
  Sum2 : Sum  Inputs=+--  InputSameDT=on  SaturateOnIntegerOverflow=on  OutDataTypeStr=Inherit: Same as first input
  Switch : Switch  Commented=on  Criteria=u2 > Threshold  SaturateOnIntegerOverflow=off  InputSameDT=off
  emission_in : Gain  Gain=emission_in  SaturateOnIntegerOverflow=on  OutDataTypeStr=Inherit: Same as input  ParamDataTypeStr=Inherit: Same as input
  lewis : Gain  Commented=on  Gain=0.000000007  SaturateOnIntegerOverflow=on  OutDataTypeStr=Inherit: Same as input  ParamDataTypeStr=Inherit: Same as input
  nomassflow : Constant  Value=0
  ps_l : Fcn  Commented=on  Expr=610.0*exp(17.08*(u)/(234.2+(u)))
  ps_s_l : Fcn  Commented=on  Expr=610.0*exp(17.08*(u)/(234.2+(u)))
  sigma : Constant  Value=5.67e-8
  sun_neg1 : Gain  Gain=-1  SaturateOnIntegerOverflow=on  OutDataTypeStr=Inherit: Same as input  ParamDataTypeStr=Inherit: Same as input
  view_factor : Gain  Gain=view_factor  SaturateOnIntegerOverflow=on  OutDataTypeStr=Inherit: Same as input  ParamDataTypeStr=Inherit: Same as input
  wallsurface1 : Gain  Commented=on  Gain=wallsurface  SaturateOnIntegerOverflow=on  OutDataTypeStr=Inherit: Same as input  ParamDataTypeStr=Inherit: Same as input
  wallsurface2 : Gain  Gain=wallsurface  SaturateOnIntegerOverflow=on  OutDataTypeStr=Inherit: Same as input  ParamDataTypeStr=Inherit: Same as input
  wallsurface3 : Gain  Gain=wallsurface  SaturateOnIntegerOverflow=on  OutDataTypeStr=Inherit: Same as input  ParamDataTypeStr=Inherit: Same as input
  wallsurface4 : Gain  Gain=wallsurface  SaturateOnIntegerOverflow=on  OutDataTypeStr=Inherit: Same as input  ParamDataTypeStr=Inherit: Same as input
  x2RelHum_UIBK : carnot/Basic/Material_Properties/x2RelHum  Commented=on
      settings: SourceProductName=Carnot
  qdots : Outport  InitialOutput=0  VectorParamsAs1DForOutWhenUnconnected=off
  "[S]" : Outport  Port=2  InitialOutput=0  VectorParamsAs1DForOutWhenUnconnected=off
  alpha_c : Outport  Port=3  InitialOutput=0  VectorParamsAs1DForOutWhenUnconnected=off
  phi_i_1/100 : Outport  Port=4  InitialOutput=0  VectorParamsAs1DForOutWhenUnconnected=off
  wires:
  1/wallsurface/1 -> Sum2/1
  Qdot sol/1 -> 1/wallsurface/1
  Fcn/1 -> Product1/2, alpha_c/1  "hc"
  Product1/1 -> wallsurface2/1, Sum2/2  "qdotc"
  Mux2/1 -> Fcn/1
  Bus Selector/2 -> Mux3/2  "<Tr>"
  Sum/1 -> Product1/1  "dTc"
  Ts/1 -> Mux2/1, Mux3/1, ps_s_l/1, Sum/1  "Ts"
  Product/1 -> Sum2/3, wallsurface3/1  "qdotr"
  emission_in/1 -> view_factor/1
  Bus Selector/1 -> x2RelHum_UIBK/1, ps_l/1, Mux2/2, Sum/2  "<Tc>"
  AIB/1 -> Bus Selector/1
  Sum2/1 -> wallsurface4/1, qdots/1
  sigma/1 -> emission_in/1
  Mux3/1 -> Fcn1/1
  Fcn1/1 -> Product/2
  x2RelHum_UIBK/1 -> Gain2/1
  Bus Selector/3 -> x2RelHum_UIBK/2  "<p>"
  Bus Selector/4 -> x2RelHum_UIBK/3  "<x_H2O>"
  Gain2/1 -> phi_i_1/100/1, Product2/1
  lewis/1 -> wallsurface1/1
  ps_l/1 -> Product2/2
  ps_s_l/1 -> Product3/2
  Product3/1 -> Add/1
  Product2/1 -> Add/2
  Add/1 -> lewis/1
  phis/1 -> Switch/2, Product3/1
  view_factor/1 -> Product/1
  wallsurface1/1 -> Switch/1
  nomassflow/1 -> Bus Assignment2/5, Switch/3
  S_initialize/1 -> Bus Assignment2/1
  wallsurface2/1 -> Bus Assignment2/2  "Qdotc"
  wallsurface3/1 -> Bus Assignment2/3  "Qdotr"
  sun_neg1/1 -> Bus Assignment2/4
  wallsurface4/1 -> sun_neg1/1  "Qdotr"
  Bus Assignment2/1 -> "[S]"/1

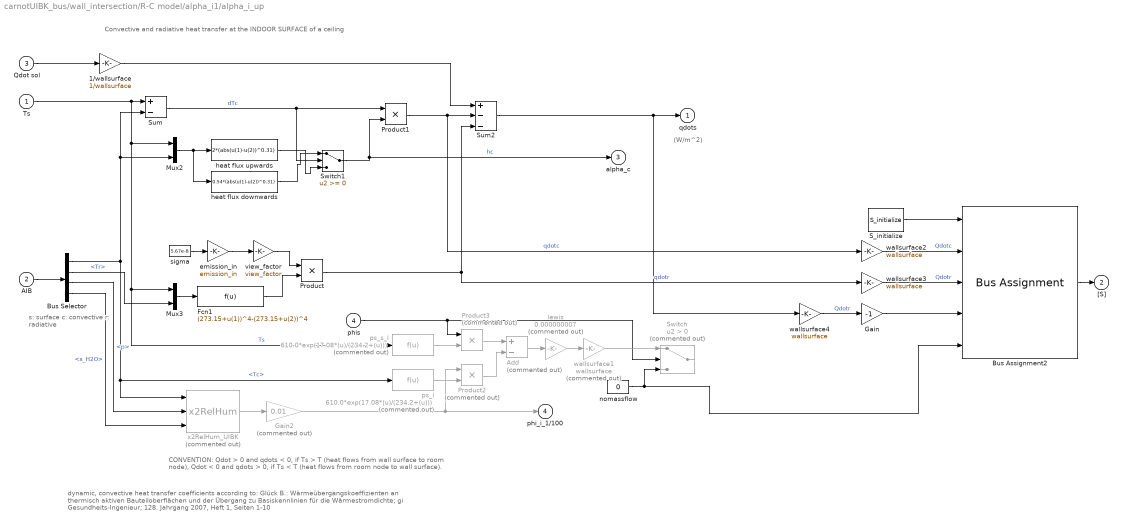
== system carnotUIBK_bus/wall_intersection/R-C model/alpha_i1/alpha_i_up ==
  note: dynamic, convective heat transfer coefficients according to: Glück B.: Wärmeübergangskoeffizienten an thermisch aktiven Bauteiloberflächen
      | und der Übergang zu Basiskennlinien für die Wärmestromdichte; gi Gesundheits-Ingenieur; 128. Jahrgang 2007, Heft 1, Seiten 1-10
  note: s: surface
      | c: convective
      | r: radiative
  note: CONVENTION:
      | Qdot > 0 and qdots < 0, if Ts > T (heat flows from wall surface to room node),
      | Qdot < 0 and qdots > 0, if Ts < T (heat flows from room node to wall surface).
  note: Convective and radiative heat transfer at the INDOOR SURFACE of a ceiling
  note: (W/m^2)
  Ts : Inport
  AIB : Inport  Port=2
  Qdot sol : Inport  Port=3
  phis : Inport  Port=4
  1/wallsurface : Gain  Gain=1/wallsurface  SaturateOnIntegerOverflow=on  OutDataTypeStr=Inherit: Same as input  ParamDataTypeStr=Inherit: Same as input
  Add : Sum  Commented=on  Inputs=+-
  Bus Assignment2 : BusAssignment  AssignedSignals=Qdotc,Qdotr,Qdot_T_neighbour,mdot_H2O
  Bus Selector : BusSelector  OutputSignals=Tc,Tr,p,x_H2O
  Fcn1 : Fcn  Expr=(273.15+u(1))^4-(273.15+u(2))^4
  Gain : Gain  Gain=-1
  Gain2 : Gain  Commented=on  Gain=0.01
  Mux2 : Mux  Inputs=2
  Mux3 : Mux  Inputs=2
  Product : Product  InputSameDT=on  RndMeth=Zero  SaturateOnIntegerOverflow=on  OutDataTypeStr=Inherit: Same as first input
  Product1 : Product  InputSameDT=on  RndMeth=Zero  SaturateOnIntegerOverflow=on  OutDataTypeStr=Inherit: Same as first input
  Product2 : Product  Commented=on  RndMeth=Zero
  Product3 : Product  Commented=on  RndMeth=Zero
  S_initialize : $bdroot/general/S_initialize  SystemSampleTime=-1  VariantActivationTime=update diagram  AllowFlexibleInterface=on  Latency=0  AutoFrameSizeCalculation=off
  Sum : Sum  Inputs=+-  InputSameDT=on  SaturateOnIntegerOverflow=on  OutDataTypeStr=Inherit: Same as first input
  Sum2 : Sum  Inputs=+--  InputSameDT=on  SaturateOnIntegerOverflow=on  OutDataTypeStr=Inherit: Same as first input
  Switch : Switch  Commented=on  Criteria=u2 > Threshold  SaturateOnIntegerOverflow=off  InputSameDT=off
  Switch1 : Switch  SaturateOnIntegerOverflow=off  InputSameDT=off
  emission_in : Gain  Gain=emission_in  SaturateOnIntegerOverflow=on  OutDataTypeStr=Inherit: Same as input  ParamDataTypeStr=Inherit: Same as input
  heat flux downwards : Fcn  Expr=0.54*(abs(u(1)-u(2))^0.31)
  heat flux upwards : Fcn  Expr=2*(abs(u(1)-u(2))^0.31)
  lewis : Gain  Commented=on  Gain=0.000000007  SaturateOnIntegerOverflow=on  OutDataTypeStr=Inherit: Same as input  ParamDataTypeStr=Inherit: Same as input
  nomassflow : Constant  Value=0
  ps_l : Fcn  Commented=on  Expr=610.0*exp(17.08*(u)/(234.2+(u)))
  ps_s_l : Fcn  Commented=on  Expr=610.0*exp(17.08*(u)/(234.2+(u)))
  sigma : Constant  Value=5.67e-8
  view_factor : Gain  Gain=view_factor  SaturateOnIntegerOverflow=on  OutDataTypeStr=Inherit: Same as input  ParamDataTypeStr=Inherit: Same as input
  wallsurface1 : Gain  Commented=on  Gain=wallsurface  SaturateOnIntegerOverflow=on  OutDataTypeStr=Inherit: Same as input  ParamDataTypeStr=Inherit: Same as input
  wallsurface2 : Gain  Gain=wallsurface  SaturateOnIntegerOverflow=on  OutDataTypeStr=Inherit: Same as input  ParamDataTypeStr=Inherit: Same as input
  wallsurface3 : Gain  Gain=wallsurface  SaturateOnIntegerOverflow=on  OutDataTypeStr=Inherit: Same as input  ParamDataTypeStr=Inherit: Same as input
  wallsurface4 : Gain  Gain=wallsurface  SaturateOnIntegerOverflow=on  OutDataTypeStr=Inherit: Same as input  ParamDataTypeStr=Inherit: Same as input
  x2RelHum_UIBK : carnot/Basic/Material_Properties/x2RelHum  Commented=on
      settings: SourceProductName=Carnot
  qdots : Outport  InitialOutput=0  VectorParamsAs1DForOutWhenUnconnected=off
  "[S]" : Outport  Port=2  InitialOutput=0  VectorParamsAs1DForOutWhenUnconnected=off
  alpha_c : Outport  Port=3  InitialOutput=0  VectorParamsAs1DForOutWhenUnconnected=off
  phi_i_1/100 : Outport  Port=4  InitialOutput=0  VectorParamsAs1DForOutWhenUnconnected=off
  wires:
  heat flux downwards/1 -> Switch1/1
  heat flux upwards/1 -> Switch1/3
  Sum/1 -> Product1/1, Switch1/2  "dTc"
  1/wallsurface/1 -> Sum2/1
  Qdot sol/1 -> 1/wallsurface/1
  Switch1/1 -> alpha_c/1, Product1/2  "hc"
  Product1/1 -> wallsurface2/1, Sum2/2  "qdotc"
  Mux2/1 -> heat flux upwards/1, heat flux downwards/1
  Bus Selector/2 -> Mux3/2  "<Tr>"
  Ts/1 -> Mux2/1, Mux3/1, ps_s_l/1, Sum/1  "Ts"
  Product/1 -> Sum2/3, wallsurface3/1  "qdotr"
  emission_in/1 -> view_factor/1
  Bus Selector/1 -> x2RelHum_UIBK/1, ps_l/1, Mux2/2, Sum/2  "<Tc>"
  AIB/1 -> Bus Selector/1
  Sum2/1 -> wallsurface4/1, qdots/1
  sigma/1 -> emission_in/1
  Mux3/1 -> Fcn1/1
  Fcn1/1 -> Product/2
  x2RelHum_UIBK/1 -> Gain2/1
  Bus Selector/3 -> x2RelHum_UIBK/2  "<p>"
  Bus Selector/4 -> x2RelHum_UIBK/3  "<x_H2O>"
  Gain2/1 -> phi_i_1/100/1, Product2/1
  lewis/1 -> wallsurface1/1
  ps_l/1 -> Product2/2
  ps_s_l/1 -> Product3/2
  Product3/1 -> Add/1
  Product2/1 -> Add/2
  Add/1 -> lewis/1
  phis/1 -> Switch/2, Product3/1
  view_factor/1 -> Product/1
  wallsurface1/1 -> Switch/1
  nomassflow/1 -> Bus Assignment2/5, Switch/3
  wallsurface3/1 -> Bus Assignment2/3  "Qdotr"
  wallsurface2/1 -> Bus Assignment2/2  "Qdotc"
  S_initialize/1 -> Bus Assignment2/1
  Bus Assignment2/1 -> "[S]"/1
  wallsurface4/1 -> Gain/1  "Qdotr"
  Gain/1 -> Bus Assignment2/4
